simulink model "BiegeMaschineAllein_2"  (R2013b)
settings: Solver=ode45  StartTime=0.0  StopTime=10  RelTol=1e-3
libraries: simulink x8
settings Model: Creator=taprudho  LastModifiedBy=daniw
settings DataIOCC: SignalLoggingSaveFormat=ModelDataLogs
settings OptimizationCC: ExpressionDepthLimit=2147483647  SimCompilerOptimization=off
settings DebuggingCC: FcnCallInpInsideContextMsg=UseLocalSettings  FrameProcessingCompatibilityMsg=error  AllowSymbolicDim=off  StateNameClashWarn=warning  StrictBusMsg=Warning
settings SFSimCC: SimParseCustomCode=off
settings RTWCC: RTWCompilerOptimization=off
settings GRTTargetCC: TargetLangStandard=C89/C90 (ANSI)  CodeReplacementLibrary=None  CombineOutputUpdateFcns=off  CPPClassGenCompliant=on  GRTInterface=on
settings ConfigComp: CovMetricSettings=dw  CovHtmlReporting=on  CovSaveCumulativeToWorkspaceVar=on  CovSaveSingleToWorkspaceVar=on  CovModelRefEnable=Off  CovExternalEMLEnable=off  CovSFcnEnable=off

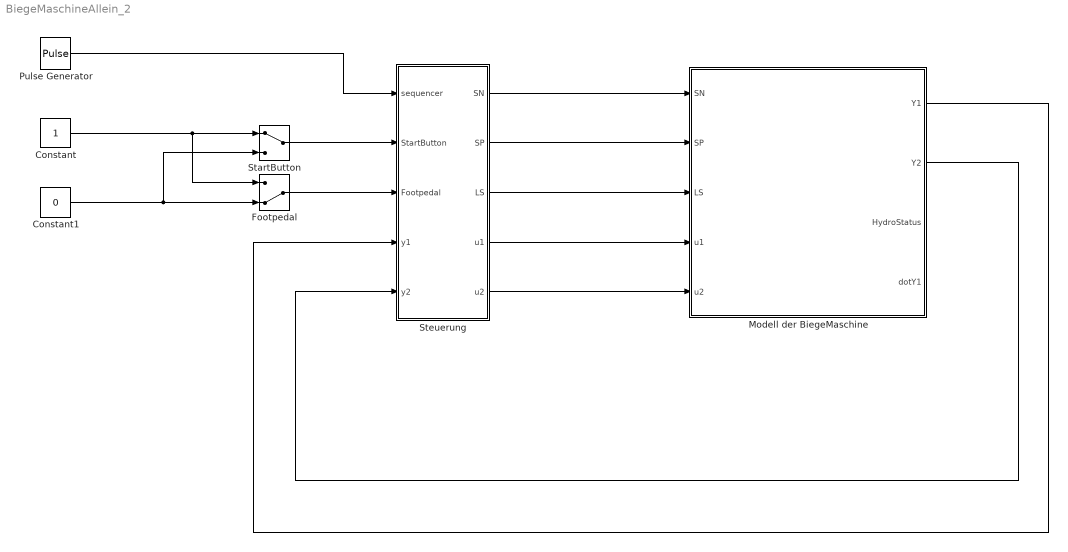
== system BiegeMaschineAllein_2 ==
  Constant : Constant
  Constant1 : Constant  Value=0
  Footpedal : ManualSwitch  CurrentSetting=0
  Modell der BiegeMaschine : Subsystem
  Pulse Generator : DiscretePulseGenerator  Period=10  PulseWidth=5  SampleTime=0.001
  StartButton : ManualSwitch
  Steuerung : Subsystem
  wires:
  Modell der BiegeMaschine/1(Y1) -> Steuerung/4(y1)
  Modell der BiegeMaschine/2(Y2) -> Steuerung/5(y2)
  Steuerung/2(SP) -> Modell der BiegeMaschine/2(SP)
  Steuerung/4(u1) -> Modell der BiegeMaschine/4(u1)
  Steuerung/5(u2) -> Modell der BiegeMaschine/5(u2)
  Steuerung/3(LS) -> Modell der BiegeMaschine/3(LS)
  Steuerung/1(SN) -> Modell der BiegeMaschine/1(SN)
  StartButton/1 -> Steuerung/2(StartButton)
  Footpedal/1 -> Steuerung/3(Footpedal)
  Constant/1 -> Footpedal/1, StartButton/1
  Constant1/1 -> StartButton/2, Footpedal/2
  Pulse Generator/1 -> Steuerung/1(sequencer)

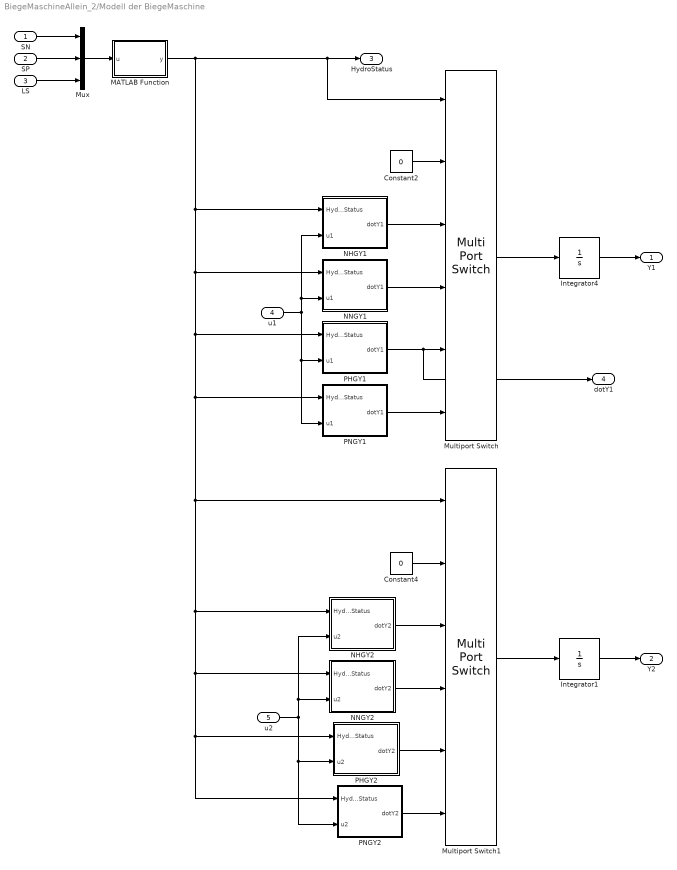
== system BiegeMaschineAllein_2/Modell der BiegeMaschine ==
  SN : Inport
  SP : Inport  Port=2
  LS : Inport  Port=3
  u1 : Inport  Port=4
  u2 : Inport  Port=5
  Constant2 : Constant  Value=0
  Constant4 : Constant  Value=0
  Integrator1 : Integrator
  Integrator4 : Integrator
  MATLAB Function : MATLAB Function  TreatAsAtomicUnit=on
  Multiport Switch : MultiPortSwitch  Inputs=5
  Multiport Switch1 : MultiPortSwitch  Inputs=5
  Mux : Mux  Inputs=3
  NHGY1 : Subsystem
  NHGY2 : Subsystem
  NNGY1 : Subsystem
  NNGY2 : Subsystem
  PHGY1 : Subsystem
  PHGY2 : Subsystem
  PNGY1 : Subsystem
  PNGY2 : Subsystem
  Y1 : Outport
  Y2 : Outport  Port=2
  HydroStatus : Outport  Port=3
  dotY1 : Outport  Port=4
  wires:
  SN/1 -> Mux/1
  SP/1 -> Mux/2
  LS/1 -> Mux/3
  Mux/1 -> MATLAB Function/1(u)
  MATLAB Function/1(y) -> Multiport Switch/1, HydroStatus/1, NHGY1/1(HydroStatus), NNGY1/1(HydroStatus), PHGY1/1(HydroStatus), Multiport Switch1/1, NHGY2/1(HydroStatus), NNGY2/1(HydroStatus), PHGY2/1(HydroStatus), PNGY2/1(HydroStatus), PNGY1/1(HydroStatus)
  NHGY1/1(dotY1) -> Multiport Switch/3
  NNGY1/1(dotY1) -> Multiport Switch/4
  PHGY1/1(dotY1) -> Multiport Switch/5, dotY1/1
  PNGY1/1(dotY1) -> Multiport Switch/6
  Constant2/1 -> Multiport Switch/2
  Multiport Switch/1 -> Integrator4/1
  Integrator4/1 -> Y1/1
  Constant4/1 -> Multiport Switch1/2
  NHGY2/1(dotY2) -> Multiport Switch1/3
  NNGY2/1(dotY2) -> Multiport Switch1/4
  PHGY2/1(dotY2) -> Multiport Switch1/5
  u2/1 -> NHGY2/2(u2), NNGY2/2(u2), PHGY2/2(u2), PNGY2/2(u2)
  Multiport Switch1/1 -> Integrator1/1
  Integrator1/1 -> Y2/1
  PNGY2/1(dotY2) -> Multiport Switch1/6
  u1/1 -> NHGY1/2(u1), NNGY1/2(u1), PHGY1/2(u1), PNGY1/2(u1)

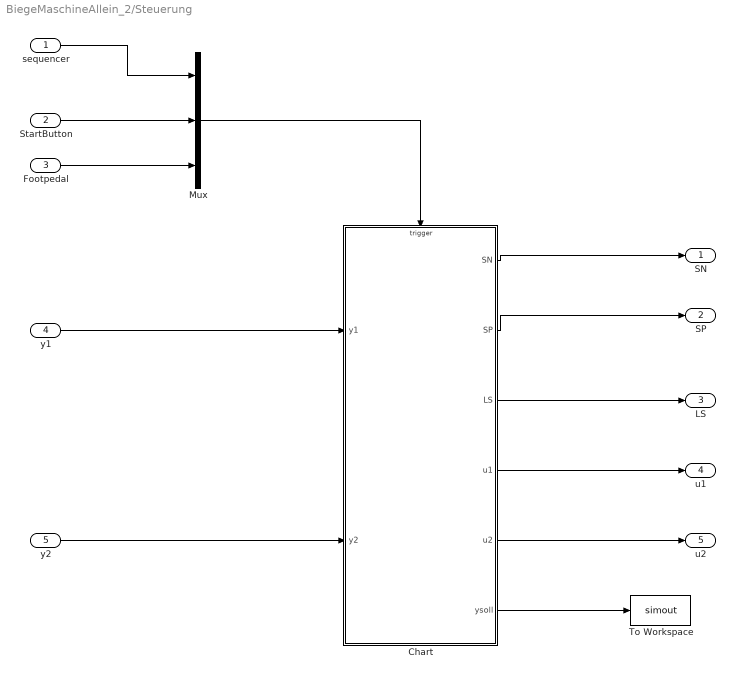
== system BiegeMaschineAllein_2/Steuerung ==
  sequencer : Inport
  StartButton : Inport  Port=2
  Footpedal : Inport  Port=3
  y1 : Inport  Port=4
  y2 : Inport  Port=5
  Chart : Stateflow chart  TreatAsAtomicUnit=on
  Mux : Mux  Inputs=3
  To Workspace : ToWorkspace  VariableName=simout  SampleTime=-1  SaveFormat=Timeseries
  SN : Outport
  SP : Outport  Port=2
  LS : Outport  Port=3
  u1 : Outport  Port=4
  u2 : Outport  Port=5
  wires:
  StartButton/1 -> Mux/2
  Mux/1 -> Chart/Trigger
  Footpedal/1 -> Mux/3
  y1/1 -> Chart/1(y1)
  y2/1 -> Chart/2(y2)
  Chart/1(SN) -> SN/1
  Chart/2(SP) -> SP/1
  Chart/3(LS) -> LS/1
  Chart/4(u1) -> u1/1
  sequencer/1 -> Mux/1
  Chart/5(u2) -> u2/1
  Chart/6(ysoll) -> To Workspace/1

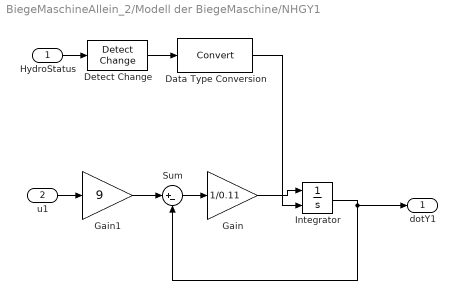
== system BiegeMaschineAllein_2/Modell der BiegeMaschine/NHGY1 ==
  HydroStatus : Inport
  u1 : Inport  Port=2
  Data Type Conversion : DataTypeConversion
  Detect Change : simulink/Logic and Bit Operations/Detect Change  vinit=0  InputProcessing=Inherited  OutDataTypeStr=boolean
  Gain : Gain  Gain=1/0.11
  Gain1 : Gain  Gain=9
  Integrator : Integrator  ExternalReset=either
  Sum : Sum  Inputs=|+-
  dotY1 : Outport
  wires:
  Gain/1 -> Integrator/1
  Sum/1 -> Gain/1
  Gain1/1 -> Sum/1
  Integrator/1 -> Sum/2, dotY1/1
  HydroStatus/1 -> Detect Change/1
  u1/1 -> Gain1/1
  Detect Change/1 -> Data Type Conversion/1
  Data Type Conversion/1 -> Integrator/2

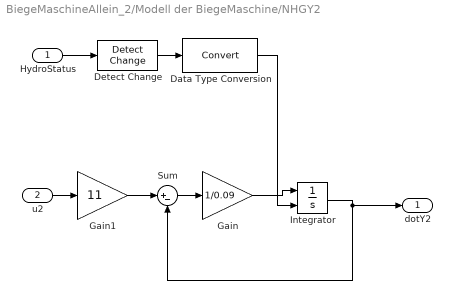
== system BiegeMaschineAllein_2/Modell der BiegeMaschine/NHGY2 ==
  HydroStatus : Inport
  u2 : Inport  Port=2
  Data Type Conversion : DataTypeConversion
  Detect Change : simulink/Logic and Bit Operations/Detect Change  vinit=0  InputProcessing=Inherited  OutDataTypeStr=uint8
  Gain : Gain  Gain=1/0.09
  Gain1 : Gain  Gain=11
  Integrator : Integrator  ExternalReset=either
  Sum : Sum  Inputs=|+-
  dotY2 : Outport
  wires:
  Gain/1 -> Integrator/1
  Sum/1 -> Gain/1
  Gain1/1 -> Sum/1
  Integrator/1 -> Sum/2, dotY2/1
  HydroStatus/1 -> Detect Change/1
  u2/1 -> Gain1/1
  Detect Change/1 -> Data Type Conversion/1
  Data Type Conversion/1 -> Integrator/2

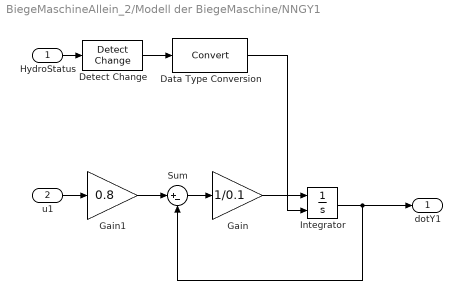
== system BiegeMaschineAllein_2/Modell der BiegeMaschine/NNGY1 ==
  HydroStatus : Inport
  u1 : Inport  Port=2
  Data Type Conversion : DataTypeConversion
  Detect Change : simulink/Logic and Bit Operations/Detect Change  vinit=0  InputProcessing=Inherited  OutDataTypeStr=uint8
  Gain : Gain  Gain=1/0.1
  Gain1 : Gain  Gain=0.8
  Integrator : Integrator  ExternalReset=either
  Sum : Sum  Inputs=|+-
  dotY1 : Outport
  wires:
  Gain/1 -> Integrator/1
  Sum/1 -> Gain/1
  Gain1/1 -> Sum/1
  Integrator/1 -> Sum/2, dotY1/1
  Detect Change/1 -> Data Type Conversion/1
  HydroStatus/1 -> Detect Change/1
  u1/1 -> Gain1/1
  Data Type Conversion/1 -> Integrator/2

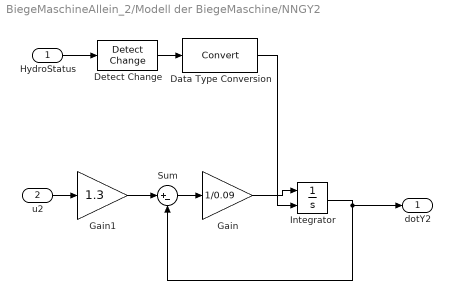
== system BiegeMaschineAllein_2/Modell der BiegeMaschine/NNGY2 ==
  HydroStatus : Inport
  u2 : Inport  Port=2
  Data Type Conversion : DataTypeConversion
  Detect Change : simulink/Logic and Bit Operations/Detect Change  vinit=0  InputProcessing=Inherited  OutDataTypeStr=uint8
  Gain : Gain  Gain=1/0.09
  Gain1 : Gain  Gain=1.3
  Integrator : Integrator  ExternalReset=either
  Sum : Sum  Inputs=|+-
  dotY2 : Outport
  wires:
  Gain/1 -> Integrator/1
  Sum/1 -> Gain/1
  Gain1/1 -> Sum/1
  Integrator/1 -> Sum/2, dotY2/1
  HydroStatus/1 -> Detect Change/1
  u2/1 -> Gain1/1
  Detect Change/1 -> Data Type Conversion/1
  Data Type Conversion/1 -> Integrator/2

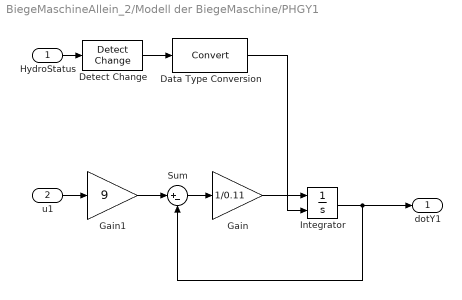
== system BiegeMaschineAllein_2/Modell der BiegeMaschine/PHGY1 ==
  HydroStatus : Inport
  u1 : Inport  Port=2
  Data Type Conversion : DataTypeConversion
  Detect Change : simulink/Logic and Bit Operations/Detect Change  vinit=0  InputProcessing=Inherited  OutDataTypeStr=uint8
  Gain : Gain  Gain=1/0.11
  Gain1 : Gain  Gain=9
  Integrator : Integrator  ExternalReset=either
  Sum : Sum  Inputs=|+-
  dotY1 : Outport
  wires:
  Gain/1 -> Integrator/1
  Sum/1 -> Gain/1
  Gain1/1 -> Sum/1
  Integrator/1 -> Sum/2, dotY1/1
  Detect Change/1 -> Data Type Conversion/1
  HydroStatus/1 -> Detect Change/1
  u1/1 -> Gain1/1
  Data Type Conversion/1 -> Integrator/2

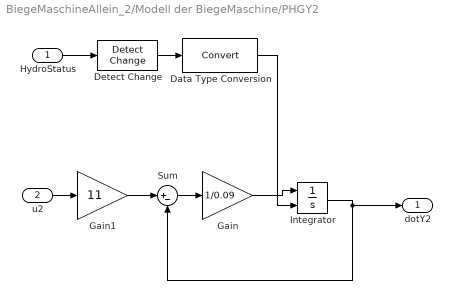
== system BiegeMaschineAllein_2/Modell der BiegeMaschine/PHGY2 ==
  HydroStatus : Inport
  u2 : Inport  Port=2
  Data Type Conversion : DataTypeConversion
  Detect Change : simulink/Logic and Bit Operations/Detect Change  vinit=0  InputProcessing=Inherited  OutDataTypeStr=uint8
  Gain : Gain  Gain=1/0.09
  Gain1 : Gain  Gain=11
  Integrator : Integrator  ExternalReset=either
  Sum : Sum  Inputs=|+-
  dotY2 : Outport
  wires:
  Gain/1 -> Integrator/1
  Sum/1 -> Gain/1
  Gain1/1 -> Sum/1
  Integrator/1 -> Sum/2, dotY2/1
  HydroStatus/1 -> Detect Change/1
  u2/1 -> Gain1/1
  Detect Change/1 -> Data Type Conversion/1
  Data Type Conversion/1 -> Integrator/2

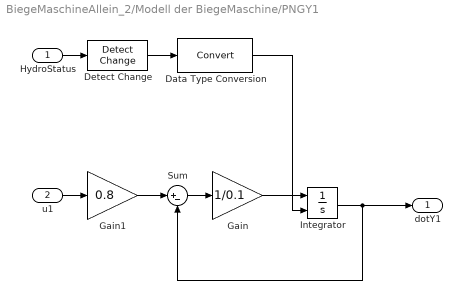
== system BiegeMaschineAllein_2/Modell der BiegeMaschine/PNGY1 ==
  HydroStatus : Inport
  u1 : Inport  Port=2
  Data Type Conversion : DataTypeConversion
  Detect Change : simulink/Logic and Bit Operations/Detect Change  vinit=0  InputProcessing=Inherited  OutDataTypeStr=uint8
  Gain : Gain  Gain=1/0.1
  Gain1 : Gain  Gain=0.8
  Integrator : Integrator  ExternalReset=either
  Sum : Sum  Inputs=|+-
  dotY1 : Outport
  wires:
  Gain/1 -> Integrator/1
  Sum/1 -> Gain/1
  Gain1/1 -> Sum/1
  Integrator/1 -> Sum/2, dotY1/1
  u1/1 -> Gain1/1
  Detect Change/1 -> Data Type Conversion/1
  Data Type Conversion/1 -> Integrator/2
  HydroStatus/1 -> Detect Change/1

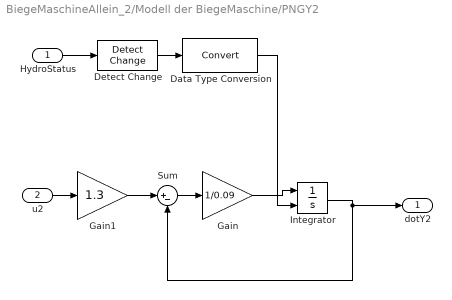
== system BiegeMaschineAllein_2/Modell der BiegeMaschine/PNGY2 ==
  HydroStatus : Inport
  u2 : Inport  Port=2
  Data Type Conversion : DataTypeConversion
  Detect Change : simulink/Logic and Bit Operations/Detect Change  vinit=0  InputProcessing=Inherited  OutDataTypeStr=uint8
  Gain : Gain  Gain=1/0.09
  Gain1 : Gain  Gain=1.3
  Integrator : Integrator  ExternalReset=either
  Sum : Sum  Inputs=|+-
  dotY2 : Outport
  wires:
  Gain/1 -> Integrator/1
  Sum/1 -> Gain/1
  Gain1/1 -> Sum/1
  Integrator/1 -> Sum/2, dotY2/1
  HydroStatus/1 -> Detect Change/1
  u2/1 -> Gain1/1
  Detect Change/1 -> Data Type Conversion/1
  Data Type Conversion/1 -> Integrator/2

== matlab function BiegeMaschineAllein_2/Modell der BiegeMaschine/Embedded MATLAB Function ==
  data: u input; y output
function y  = fcn(u)
% This block supports the Embedded MATLAB subset.
% See the help menu for details. 

% Inputs
SN = u(1);
SP = u(2);
LS = u(3);

% Outputs
STOP = 1;
NHG = 2;
NNG = 3;
PHG = 4;
PNG = 5;


if ((SN > 0.7) && (SP < 0.3) && (LS < 0.3))
    y = NHG;
elseif ((SN > 0.7) && (SP < 0.3) && (LS > 0.7))
    y = NNG;
elseif ((SN < 0.3) && (SP > 0.7) && (LS < 0.3))
    y = PHG;
elseif ((SN < 0.3) && (SP > 0.7) && (LS > 0.7))
    y = PNG;    
else
    y = STOP;
end

== stateflow chart BiegeMaschineAllein_2/Steuerung/Chart ==
  state PreInit
  state Init
    entry: tk = 0.0;
    entry: [a3,a2,a1,a0] = TrajectoryPreparation(200.0,y1,2.0);
  state State2
    on every(1,sequencer): ysoll = TrajectoryComputation(a3,a2,a1,a0,tk);
    on every(1,sequencer): [u1,e1] = PID(ysoll, y1, Kp1, Ti1, Td1, Ts, e1, u1);
    on every(1,sequencer): tk = tk + 0.01;
  state Stop
    on every(1,sequencer): ysoll = 200.0;
    on every(1,sequencer): PID(ysoll,y1,Kp1,Ti1,Td1,Ts,e1,u1);
  (default) -> PreInit
  PreInit -> Init : FootpedalPressed
  Init -> State2 : after(20,sequencer)
  State2 -> Stop
  data: r function_input double; y function_input double; Kp function_input double; Ti function_input double; Td function_input double; T function_input double; e_old function_input double; ui_old function_input double; u function_output double; e function_output double; y_target_p function_input double; y_ist_p function_input double; a3p function_output double; tf_p function_input double; a2p function_output double; a1p function_output double; a0p function_output double; a3p function_input double; a2p function_input double; a1p function_input double; a0p function_input double; tkp function_input double; ysollp function_output double; y1 input; y2 input; SN output double =0; SP output double =0; LS output double =0; u1 output double =0; u2 output double =0; Kp constant double =3.0;; Y1ref constant double =55.0;; e1 local double =0; ysoll output double =0; Kp1 constant double =0.1;; Td1 constant double =0.1;; Ti1 constant double =3000;; Ts constant double =0.01;; a0 local double; a1 local double; a2 local double; a3 local double; tk local double
  events: sequencer input RISING_EDGE_EVENT; StartButtonPressed input RISING_EDGE_EVENT; FootpedalPressed input RISING_EDGE_EVENT
  function [u, e]  = PID(r,y,Kp,Ti,Td,T,e_old,ui_old):
    | function [u,e] = PID(r,y,Kp,Ti,Td,T,e_old,ui_old)
    | 
    | % Regelfehler
    | e = r-y;
    | 
    | % P Anteil
    | up = Kp*e;
    | 
    | % I Anteil (Trapezregel)
    | ui = ui_old + T/Ti*(e+e_old)/2;
    | 
    | % D Anteil (Rückwärts- Rechteckregel)
    | ud = Td * (e-e_old)/T;
    | 
    | u = up+ui+ud;
  function [a3p,a2p,a1p,a0p] = TrajectoryPreparation(y_target_p,y_ist_p,tf_p):
    | function [a3p,a2p,a1p,a0p] = TrajectoryPreparation(y_target_p,y_ist_p,tf_p)
    | 
    | a0p = y_ist_p;
    | a1p = 0.0;
    | a2p = 3*(y_target_p - y_ist_p)/(tf_p*tf_p);
    | a3p = 2*(y_ist_p - y_target_p)/(tf_p*tf_p*tf_p);
  function ysollp  = TrajectoryComputation(a3p,a2p,a1p,a0p,tkp):
    | function ysollp  = TrajectoryComputation(a3p,a2p,a1p,a0p,tkp)
    | 
    | ysollp = a3p*tkp^3+a2p*tkp^2+a1p*tkp+a0p;

== matlab function BiegeMaschineAllein_2/Modell der BiegeMaschine/MATLAB Function ==
  data: u input; y output
function y  = fcn(u)
% This block supports the Embedded MATLAB subset.
% See the help menu for details.

% Inputs
SN = u(1);
SP = u(2);
LS = u(3);

% Outputs
STOP = 1;
NHG = 2;
NNG = 3;
PHG = 4;
PNG = 5;


if ((SN > 0.7) && (SP < 0.3) && (LS < 0.3))
    y = NHG;
elseif ((SN > 0.7) && (SP < 0.3) && (LS > 0.7))
    y = NNG;
elseif ((SN < 0.3) && (SP > 0.7) && (LS < 0.3))
    y = PHG;
elseif ((SN < 0.3) && (SP > 0.7) && (LS > 0.7))
    y = PNG;   
else
    y = STOP;
end
